simulink model "A_LN"  (R2021b)
settings: Solver=VariableStepAuto  StartTime=0.0  StopTime=10.0  RelTol=1e-3
settings Model: Creator=adity  LastModifiedBy=adity

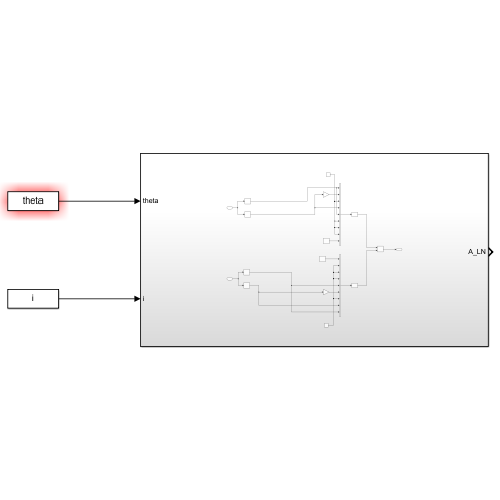
[thumbnail: Simulink's stored preview of the top-level diagram]
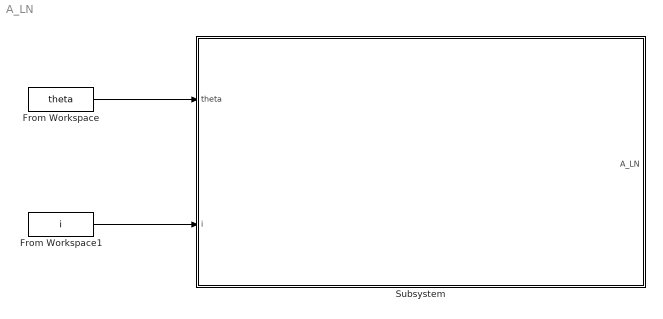
== system A_LN ==
  From Workspace : FromWorkspace  VariableName=theta
  From Workspace1 : FromWorkspace  VariableName=i
  Subsystem : Subsystem
  wires:
  From Workspace/1 -> Subsystem/1(theta)
  From Workspace1/1 -> Subsystem/2(i)

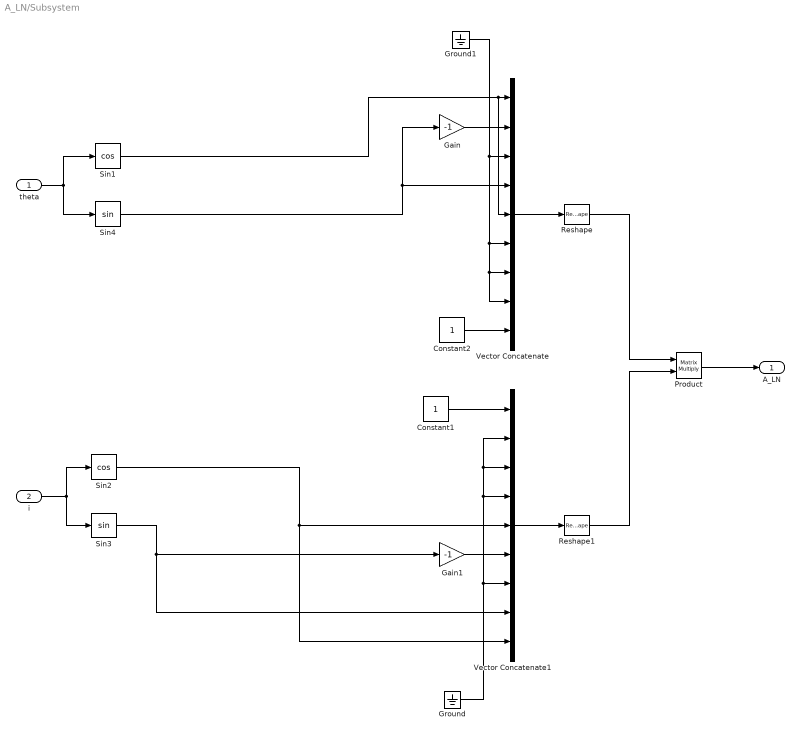
== system A_LN/Subsystem ==
  theta : Inport
  i : Inport  Port=2
  Constant1 : Constant
  Constant2 : Constant
  Gain : Gain  Gain=-1
  Gain1 : Gain  Gain=-1
  Ground : Ground
  Ground1 : Ground
  Product : Product  Multiplication=Matrix(*)
  Reshape : Reshape  OutputDimensionality=Customize  OutputDimensions=[3,3]
  Reshape1 : Reshape  OutputDimensionality=Customize  OutputDimensions=[3,3]
  Sin1 : Trigonometry  Operator=cos
  Sin2 : Trigonometry  Operator=cos
  Sin3 : Trigonometry
  Sin4 : Trigonometry
  Vector Concatenate : Concatenate  NumInputs=9
  Vector Concatenate1 : Concatenate  NumInputs=9
  A_LN : Outport
  wires:
  Vector Concatenate/1 -> Reshape/1
  Product/1 -> A_LN/1
  Reshape/1 -> Product/1
  Reshape1/1 -> Product/2
  Vector Concatenate1/1 -> Reshape1/1
  theta/1 -> Sin4/1, Sin1/1
  Sin1/1 -> Vector Concatenate/1, Vector Concatenate/5
  Gain/1 -> Vector Concatenate/2
  Sin4/1 -> Gain/1, Vector Concatenate/4
  Ground1/1 -> Vector Concatenate/6, Vector Concatenate/7, Vector Concatenate/8, Vector Concatenate/3
  Constant2/1 -> Vector Concatenate/9
  Constant1/1 -> Vector Concatenate1/1
  Ground/1 -> Vector Concatenate1/7, Vector Concatenate1/4, Vector Concatenate1/3, Vector Concatenate1/2
  i/1 -> Sin3/1, Sin2/1
  Sin2/1 -> Vector Concatenate1/9, Vector Concatenate1/5
  Gain1/1 -> Vector Concatenate1/6
  Sin3/1 -> Gain1/1, Vector Concatenate1/8
